simulink model "dsp48_firs_tb"  (Simulink 7.0)
settings: Solver=ode45  StartTime=0.0  StopTime=200  RelTol=1e-3
PreLoadFcn:
  | fir_setup_v1
StartFcn:
  | fir_setup_v1
undefined symbols (not defined in the file): A, B, C, coef, P, PCIN
libraries: xbsIndex_r4 x229, simulink x10, xbsCopyrightNotice_r4 x1, dspsrcs4 x1
(part 2 of 3)

== system dsp48_firs_tb/FIR_T1_foldx4/dsp48_1 ==
  note: Folded FIR Type1 Tap #1
  note: Tap1 - Parallel Type1 FIR filter
      | - DSP48 operation is the  function P=C+ A*B.
      | - Output routed over PCOUT.
      | - All The DSP48 internal pipeline registers are used
      | - The BCIN-BCOUT cascade is not used
      |    since larger delays are requred between stages than 2 delays
      | - The B input is configured to use 1 latency register
  ain : Inport  OutDataType=sfix(16)  OutScaling=2^0
  bin : Inport  Port=2  OutDataType=sfix(16)  OutScaling=2^0
  c : Inport  Port=3  OutDataType=sfix(16)  OutScaling=2^0
  Constant : xbsIndex_r4/Constant  arith_type=DSP48 Instruction  const=1  n_bits=1  bin_pt=0  explicit_period=off  period=1  equ=P=C+(A*B)  opselect=C + A*B  inp2=PCIN>>17  opr=+  inp1=P  carry=CIN  dbl_ovrd=off  block_type=constant
      settings: block_version=VER_STRING_GOES_HERE
  DSP2 : xbsIndex_r4/DSP48  use_b=Direct from B Port  use_op=on  use_creg=on  use_pcin=off  use_pcout=on  use_bcout=off  rst_all=off  en_all=off  pipeline_a=1  pipeline_b=1  pipeline_c=on  pipeline_p=on  pipeline_mult=on  pipeline_opmode=on  pipeline_sub=on  pipeline_carryin=on  pipeline_carryinsel=on  rst_a=off  rst_b=off  rst_c=off  rst_mult=off  rst_p=off  rst_carry_in=off  rst_ctrl=off  en_a=off  en_b=off  en_c=off  en_mult=off  en_p=off  en_carry_in=off  en_ctrl=off  dbl_ovrd=off  use_synth_model=off  xl_useadderonly=off  block_type=dsp48
      settings: xl_use_area=on  xl_area=[0, 0, 0, 0, 0, 0, 0]  block_version=VER_STRING_GOES_HERE
  Terminator1 : Terminator
  pcout : Outport  OutDataType=sfix(16)  OutScaling=2^0
  wires:
  ain/1 -> DSP2/1
  c/1 -> DSP2/3
  bin/1 -> DSP2/2
  DSP2/1 -> Terminator1/1
  DSP2/2 -> pcout/1
  Constant/1 -> DSP2/4

== system dsp48_firs_tb/FIR_T1_foldx4/dsp48_2 ==
  note: Tap2 - Parallel Type1 FIR filter
      | - DSP48 operation is the  function P=PCIN + A*B.
      | - Uses PCIN-PCOUT cascade
      | - All The DSP48 internal pipeline registers are used
      | - The BCIN-BCOUT cascade is not used
      |    since more than 2 delays are requred between stages
      | - The B input is configured to use 1 latency register
  note: Folded FIR Type1 Tap #2:n-1
  ain : Inport  OutDataType=sfix(16)  OutScaling=2^0
  bin : Inport  Port=2  OutDataType=sfix(16)  OutScaling=2^0
  pcin : Inport  Port=3  OutDataType=sfix(16)  OutScaling=2^0
  Constant : xbsIndex_r4/Constant  arith_type=DSP48 Instruction  const=1  n_bits=1  bin_pt=0  explicit_period=off  period=1  equ=P=PCIN+(A*B)  opselect=PCIN + A*B  inp2=PCIN>>17  opr=+  inp1=P  carry=CIN  dbl_ovrd=off  block_type=constant
      settings: block_version=VER_STRING_GOES_HERE
  DSP2 : xbsIndex_r4/DSP48  use_b=Direct from B Port  use_op=on  use_creg=off  use_pcin=on  use_pcout=on  use_bcout=off  rst_all=off  en_all=off  pipeline_a=1  pipeline_b=1  pipeline_c=on  pipeline_p=on  pipeline_mult=on  pipeline_opmode=on  pipeline_sub=on  pipeline_carryin=on  pipeline_carryinsel=on  rst_a=off  rst_b=off  rst_c=off  rst_mult=off  rst_p=off  rst_carry_in=off  rst_ctrl=off  en_a=off  en_b=off  en_c=off  en_mult=off  en_p=off  en_carry_in=off  en_ctrl=off  dbl_ovrd=off  use_synth_model=off  xl_useadderonly=off  block_type=dsp48
      settings: xl_use_area=on  xl_area=[0, 0, 0, 0, 0, 0, 0]  block_version=VER_STRING_GOES_HERE
  Terminator1 : Terminator
  pcout : Outport  OutDataType=sfix(16)  OutScaling=2^0
  wires:
  bin/1 -> DSP2/2
  ain/1 -> DSP2/1
  DSP2/2 -> pcout/1
  DSP2/1 -> Terminator1/1
  pcin/1 -> DSP2/3
  Constant/1 -> DSP2/4

== system dsp48_firs_tb/FIR_T1_foldx4/dsp48_3 ==
  note: Folded FIR Type1 Tap #2:n-1
  note: Tap2 - Parallel Type1 FIR filter
      | - DSP48 operation is the  function P=PCIN + A*B.
      | - Uses PCIN-PCOUT cascade
      | - All The DSP48 internal pipeline registers are used
      | - The BCIN-BCOUT cascade is not used
      |    since more than 2 delays are requred between stages
      | - The B input is configured to use 1 latency register
  ain : Inport  OutDataType=sfix(16)  OutScaling=2^0
  bin : Inport  Port=2  OutDataType=sfix(16)  OutScaling=2^0
  pcin : Inport  Port=3  OutDataType=sfix(16)  OutScaling=2^0
  Constant : xbsIndex_r4/Constant  arith_type=DSP48 Instruction  const=1  n_bits=1  bin_pt=0  explicit_period=off  period=1  equ=P=PCIN+(A*B)  opselect=PCIN + A*B  inp2=PCIN>>17  opr=+  inp1=P  carry=CIN  dbl_ovrd=off  block_type=constant
      settings: block_version=VER_STRING_GOES_HERE
  DSP2 : xbsIndex_r4/DSP48  use_b=Direct from B Port  use_op=on  use_creg=off  use_pcin=on  use_pcout=on  use_bcout=off  rst_all=off  en_all=off  pipeline_a=1  pipeline_b=1  pipeline_c=on  pipeline_p=on  pipeline_mult=on  pipeline_opmode=on  pipeline_sub=on  pipeline_carryin=on  pipeline_carryinsel=on  rst_a=off  rst_b=off  rst_c=off  rst_mult=off  rst_p=off  rst_carry_in=off  rst_ctrl=off  en_a=off  en_b=off  en_c=off  en_mult=off  en_p=off  en_carry_in=off  en_ctrl=off  dbl_ovrd=off  use_synth_model=off  xl_useadderonly=off  block_type=dsp48
      settings: xl_use_area=on  xl_area=[0, 0, 0, 0, 0, 0, 0]  block_version=VER_STRING_GOES_HERE
  Terminator1 : Terminator
  pcout : Outport  OutDataType=sfix(16)  OutScaling=2^0
  wires:
  Constant/1 -> DSP2/4
  pcin/1 -> DSP2/3
  DSP2/1 -> Terminator1/1
  DSP2/2 -> pcout/1
  ain/1 -> DSP2/1
  bin/1 -> DSP2/2

== system dsp48_firs_tb/FIR_T1_foldx4/dsp48_4 ==
  note: Tap2 - Parallel Type1 FIR filter
      | - DSP48 operation is the  function P=PCIN + A*B.
      | - Uses PCIN-PCOUT cascade
      | - All The DSP48 internal pipeline registers are used
      | - The BCIN-BCOUT cascade is not used
      |    since more than 2 delays are requred between stages
      | - The B input is configured to use 1 latency register
  note: Folded FIR Type1 Tap #2:n-1
  ain : Inport  OutDataType=sfix(16)  OutScaling=2^0
  bin : Inport  Port=2  OutDataType=sfix(16)  OutScaling=2^0
  pcin : Inport  Port=3  OutDataType=sfix(16)  OutScaling=2^0
  Constant : xbsIndex_r4/Constant  arith_type=DSP48 Instruction  const=1  n_bits=1  bin_pt=0  explicit_period=off  period=1  equ=P=PCIN+(A*B)  opselect=PCIN + A*B  inp2=PCIN>>17  opr=+  inp1=P  carry=CIN  dbl_ovrd=off  block_type=constant
      settings: block_version=VER_STRING_GOES_HERE
  DSP2 : xbsIndex_r4/DSP48  use_b=Direct from B Port  use_op=on  use_creg=off  use_pcin=on  use_pcout=on  use_bcout=off  rst_all=off  en_all=off  pipeline_a=1  pipeline_b=1  pipeline_c=on  pipeline_p=on  pipeline_mult=on  pipeline_opmode=on  pipeline_sub=on  pipeline_carryin=on  pipeline_carryinsel=on  rst_a=off  rst_b=off  rst_c=off  rst_mult=off  rst_p=off  rst_carry_in=off  rst_ctrl=off  en_a=off  en_b=off  en_c=off  en_mult=off  en_p=off  en_carry_in=off  en_ctrl=off  dbl_ovrd=off  use_synth_model=off  xl_useadderonly=off  block_type=dsp48
      settings: xl_use_area=on  xl_area=[0, 0, 0, 0, 0, 0, 0]  block_version=VER_STRING_GOES_HERE
  Terminator1 : Terminator
  pcout : Outport  OutDataType=sfix(16)  OutScaling=2^0
  wires:
  bin/1 -> DSP2/2
  ain/1 -> DSP2/1
  DSP2/2 -> pcout/1
  DSP2/1 -> Terminator1/1
  pcin/1 -> DSP2/3
  Constant/1 -> DSP2/4

== system dsp48_firs_tb/FIR_T1_foldx4/dsp48_5 ==
  note: Accumulate (ACC)
  note: ACC-  Accumulate Block
      | - DSP48 operation is one of two functions
      |   load:  P= PCIN, .
      |   accumulate: P=P+PCIN
      | - Output routed over P.
      | - All The DSP48 internal pipeline registers are used
      | - DSP48 is used because LUT based adders will not hit speed.
  pcin : Inport  OutDataType=sfix(16)  OutScaling=2^0
  load : Inport  Port=2  OutDataType=sfix(16)  OutScaling=2^0
  Constant : xbsIndex_r4/Constant  arith_type=DSP48 Instruction  const=1  n_bits=1  bin_pt=0  explicit_period=off  period=1  equ=P=PCIN+(P)  opselect=Custom  inp2=PCIN  opr=+  inp1=P  carry=0  dbl_ovrd=off  block_type=constant
      settings: block_version=VER_STRING_GOES_HERE
  Constant1 : xbsIndex_r4/Constant  arith_type=Signed (2's comp)  const=0  n_bits=18  bin_pt=0  explicit_period=on  period=1/4  equ=P=C  opselect=C  inp2=PCIN>>17  opr=+  inp1=P  carry=CIN  dbl_ovrd=off  block_type=constant
      settings: block_version=VER_STRING_GOES_HERE
  Constant2 : xbsIndex_r4/Constant  arith_type=Signed (2's comp)  const=0  n_bits=18  bin_pt=0  explicit_period=on  period=1/4  equ=P=C  opselect=C  inp2=PCIN>>17  opr=+  inp1=P  carry=CIN  dbl_ovrd=off  block_type=constant
      settings: block_version=VER_STRING_GOES_HERE
  Constant3 : xbsIndex_r4/Constant  arith_type=DSP48 Instruction  const=1  n_bits=1  bin_pt=0  explicit_period=off  period=1  equ=P=PCIN  opselect=Custom  inp2=PCIN  opr=+  inp1=0  carry=0  dbl_ovrd=off  block_type=constant
      settings: block_version=VER_STRING_GOES_HERE
  DSP48 : xbsIndex_r4/DSP48  use_b=Direct from B Port  use_op=on  use_creg=off  use_pcin=on  use_pcout=off  use_bcout=off  rst_all=off  en_all=off  pipeline_a=1  pipeline_b=1  pipeline_c=on  pipeline_p=on  pipeline_mult=on  pipeline_opmode=on  pipeline_sub=on  pipeline_carryin=on  pipeline_carryinsel=on  rst_a=off  rst_b=off  rst_c=off  rst_mult=off  rst_p=off  rst_carry_in=off  rst_ctrl=off  en_a=off  en_b=off  en_c=off  en_mult=off  en_p=off  en_carry_in=off  en_ctrl=off  dbl_ovrd=off  use_synth_model=off  xl_useadderonly=off  block_type=dsp48
      settings: xl_use_area=on  xl_area=[0, 0, 0, 0, 0, 0, 0]  block_version=VER_STRING_GOES_HERE
  Mux1 : xbsIndex_r4/Mux  inputs=2  en=off  latency=0  precision=Full  arith_type=Unsigned  n_bits=48  bin_pt=0  quantization=Truncate  overflow=Wrap  dbl_ovrd=off  block_type=mux
      settings: xl_area=[0, 0, 0, 0, 0, 0, 0]  block_version=VER_STRING_GOES_HERE
  out : Outport  OutDataType=sfix(16)  OutScaling=2^0
  wires:
  Constant2/1 -> DSP48/2
  Constant1/1 -> DSP48/1
  DSP48/1 -> out/1
  load/1 -> Mux1/1
  pcin/1 -> DSP48/3
  Mux1/1 -> DSP48/4
  Constant3/1 -> Mux1/3
  Constant/1 -> Mux1/2

== system dsp48_firs_tb/FIR_T1x16/fir_next1 ==
  note: Tap1 - Parallel Type1 FIR filter
      | - DSP48 operation is the  function P=PCIN + A*B.
      | - Output routed over PCOUT.
      | - All The DSP48 internal pipeline registers are used
      | - The BCIN-BCOUT cascade is used
      | - The B input is configured to use 2 latency registers
  note: Parallel FIR Type2 Tap #2:n-1
  ain : Inport  OutDataType=sfix(16)  OutScaling=2^0
  bcin : Inport  Port=2  OutDataType=sfix(16)  OutScaling=2^0
  pcin : Inport  Port=3  OutDataType=sfix(16)  OutScaling=2^0
  Constant : xbsIndex_r4/Constant  arith_type=DSP48 Instruction  const=1  n_bits=1  bin_pt=0  explicit_period=off  period=1  equ=P=PCIN+(A*B)  opselect=PCIN + A*B  inp2=PCIN>>17  opr=+  inp1=P  carry=CIN  dbl_ovrd=off  block_type=constant
      settings: block_version=VER_STRING_GOES_HERE
  DSP48 : xbsIndex_r4/DSP48  use_b=Cascaded from BCIN Port  use_op=on  use_creg=off  use_pcin=on  use_pcout=on  use_bcout=on  rst_all=off  en_all=off  pipeline_a=1  pipeline_b=2  pipeline_c=on  pipeline_p=on  pipeline_mult=on  pipeline_opmode=on  pipeline_sub=on  pipeline_carryin=on  pipeline_carryinsel=on  rst_a=off  rst_b=off  rst_c=off  rst_mult=off  rst_p=off  rst_carry_in=off  rst_ctrl=off  en_a=off  en_b=off  en_c=off  en_mult=off  en_p=off  en_carry_in=off  en_ctrl=off  dbl_ovrd=off  use_synth_model=off  xl_useadderonly=off  block_type=dsp48
      settings: xl_use_area=on  xl_area=[0, 0, 0, 0, 0, 0, 0]  block_version=VER_STRING_GOES_HERE
  Terminator1 : Terminator
  bcout : Outport  OutDataType=sfix(16)  OutScaling=2^0
  pcout : Outport  Port=2  OutDataType=sfix(16)  OutScaling=2^0
  wires:
  bcin/1 -> DSP48/2
  ain/1 -> DSP48/1
  DSP48/3 -> pcout/1
  DSP48/2 -> bcout/1
  DSP48/1 -> Terminator1/1
  pcin/1 -> DSP48/3
  Constant/1 -> DSP48/4

== system dsp48_firs_tb/FIR_T1x16/fir_next10 ==
  note: Parallel FIR Type2 Tap #2:n-1
  note: Tap1 - Parallel Type1 FIR filter
      | - DSP48 operation is the  function P=PCIN + A*B.
      | - Output routed over PCOUT.
      | - All The DSP48 internal pipeline registers are used
      | - The BCIN-BCOUT cascade is used
      | - The B input is configured to use 2 latency registers
  ain : Inport  OutDataType=sfix(16)  OutScaling=2^0
  bcin : Inport  Port=2  OutDataType=sfix(16)  OutScaling=2^0
  pcin : Inport  Port=3  OutDataType=sfix(16)  OutScaling=2^0
  Constant : xbsIndex_r4/Constant  arith_type=DSP48 Instruction  const=1  n_bits=1  bin_pt=0  explicit_period=off  period=1  equ=P=PCIN+(A*B)  opselect=PCIN + A*B  inp2=PCIN>>17  opr=+  inp1=P  carry=CIN  dbl_ovrd=off  block_type=constant
      settings: block_version=VER_STRING_GOES_HERE
  DSP48 : xbsIndex_r4/DSP48  use_b=Cascaded from BCIN Port  use_op=on  use_creg=off  use_pcin=on  use_pcout=on  use_bcout=on  rst_all=off  en_all=off  pipeline_a=1  pipeline_b=2  pipeline_c=on  pipeline_p=on  pipeline_mult=on  pipeline_opmode=on  pipeline_sub=on  pipeline_carryin=on  pipeline_carryinsel=on  rst_a=off  rst_b=off  rst_c=off  rst_mult=off  rst_p=off  rst_carry_in=off  rst_ctrl=off  en_a=off  en_b=off  en_c=off  en_mult=off  en_p=off  en_carry_in=off  en_ctrl=off  dbl_ovrd=off  use_synth_model=off  xl_useadderonly=off  block_type=dsp48
      settings: xl_use_area=on  xl_area=[0, 0, 0, 0, 0, 0, 0]  block_version=VER_STRING_GOES_HERE
  Terminator1 : Terminator
  bcout : Outport  OutDataType=sfix(16)  OutScaling=2^0
  pcout : Outport  Port=2  OutDataType=sfix(16)  OutScaling=2^0
  wires:
  Constant/1 -> DSP48/4
  pcin/1 -> DSP48/3
  DSP48/1 -> Terminator1/1
  DSP48/2 -> bcout/1
  DSP48/3 -> pcout/1
  ain/1 -> DSP48/1
  bcin/1 -> DSP48/2

== system dsp48_firs_tb/FIR_T1x16/fir_next11 ==
  note: Tap1 - Parallel Type1 FIR filter
      | - DSP48 operation is the  function P=PCIN + A*B.
      | - Output routed over PCOUT.
      | - All The DSP48 internal pipeline registers are used
      | - The BCIN-BCOUT cascade is used
      | - The B input is configured to use 2 latency registers
  note: Parallel FIR Type2 Tap #2:n-1
  ain : Inport  OutDataType=sfix(16)  OutScaling=2^0
  bcin : Inport  Port=2  OutDataType=sfix(16)  OutScaling=2^0
  pcin : Inport  Port=3  OutDataType=sfix(16)  OutScaling=2^0
  Constant : xbsIndex_r4/Constant  arith_type=DSP48 Instruction  const=1  n_bits=1  bin_pt=0  explicit_period=off  period=1  equ=P=PCIN+(A*B)  opselect=PCIN + A*B  inp2=PCIN>>17  opr=+  inp1=P  carry=CIN  dbl_ovrd=off  block_type=constant
      settings: block_version=VER_STRING_GOES_HERE
  DSP48 : xbsIndex_r4/DSP48  use_b=Cascaded from BCIN Port  use_op=on  use_creg=off  use_pcin=on  use_pcout=on  use_bcout=on  rst_all=off  en_all=off  pipeline_a=1  pipeline_b=2  pipeline_c=on  pipeline_p=on  pipeline_mult=on  pipeline_opmode=on  pipeline_sub=on  pipeline_carryin=on  pipeline_carryinsel=on  rst_a=off  rst_b=off  rst_c=off  rst_mult=off  rst_p=off  rst_carry_in=off  rst_ctrl=off  en_a=off  en_b=off  en_c=off  en_mult=off  en_p=off  en_carry_in=off  en_ctrl=off  dbl_ovrd=off  use_synth_model=off  xl_useadderonly=off  block_type=dsp48
      settings: xl_use_area=on  xl_area=[0, 0, 0, 0, 0, 0, 0]  block_version=VER_STRING_GOES_HERE
  Terminator1 : Terminator
  bcout : Outport  OutDataType=sfix(16)  OutScaling=2^0
  pcout : Outport  Port=2  OutDataType=sfix(16)  OutScaling=2^0
  wires:
  bcin/1 -> DSP48/2
  ain/1 -> DSP48/1
  DSP48/3 -> pcout/1
  DSP48/2 -> bcout/1
  DSP48/1 -> Terminator1/1
  pcin/1 -> DSP48/3
  Constant/1 -> DSP48/4

== system dsp48_firs_tb/FIR_T1x16/fir_next12 ==
  note: Parallel FIR Type2 Tap #2:n-1
  note: Tap1 - Parallel Type1 FIR filter
      | - DSP48 operation is the  function P=PCIN + A*B.
      | - Output routed over PCOUT.
      | - All The DSP48 internal pipeline registers are used
      | - The BCIN-BCOUT cascade is used
      | - The B input is configured to use 2 latency registers
  ain : Inport  OutDataType=sfix(16)  OutScaling=2^0
  bcin : Inport  Port=2  OutDataType=sfix(16)  OutScaling=2^0
  pcin : Inport  Port=3  OutDataType=sfix(16)  OutScaling=2^0
  Constant : xbsIndex_r4/Constant  arith_type=DSP48 Instruction  const=1  n_bits=1  bin_pt=0  explicit_period=off  period=1  equ=P=PCIN+(A*B)  opselect=PCIN + A*B  inp2=PCIN>>17  opr=+  inp1=P  carry=CIN  dbl_ovrd=off  block_type=constant
      settings: block_version=VER_STRING_GOES_HERE
  DSP48 : xbsIndex_r4/DSP48  use_b=Cascaded from BCIN Port  use_op=on  use_creg=off  use_pcin=on  use_pcout=on  use_bcout=on  rst_all=off  en_all=off  pipeline_a=1  pipeline_b=2  pipeline_c=on  pipeline_p=on  pipeline_mult=on  pipeline_opmode=on  pipeline_sub=on  pipeline_carryin=on  pipeline_carryinsel=on  rst_a=off  rst_b=off  rst_c=off  rst_mult=off  rst_p=off  rst_carry_in=off  rst_ctrl=off  en_a=off  en_b=off  en_c=off  en_mult=off  en_p=off  en_carry_in=off  en_ctrl=off  dbl_ovrd=off  use_synth_model=off  xl_useadderonly=off  block_type=dsp48
      settings: xl_use_area=on  xl_area=[0, 0, 0, 0, 0, 0, 0]  block_version=VER_STRING_GOES_HERE
  Terminator1 : Terminator
  bcout : Outport  OutDataType=sfix(16)  OutScaling=2^0
  pcout : Outport  Port=2  OutDataType=sfix(16)  OutScaling=2^0
  wires:
  Constant/1 -> DSP48/4
  pcin/1 -> DSP48/3
  DSP48/1 -> Terminator1/1
  DSP48/2 -> bcout/1
  DSP48/3 -> pcout/1
  ain/1 -> DSP48/1
  bcin/1 -> DSP48/2

== system dsp48_firs_tb/FIR_T1x16/fir_next13 ==
  note: Tap1 - Parallel Type1 FIR filter
      | - DSP48 operation is the  function P=PCIN + A*B.
      | - Output routed over PCOUT.
      | - All The DSP48 internal pipeline registers are used
      | - The BCIN-BCOUT cascade is used
      | - The B input is configured to use 2 latency registers
  note: Parallel FIR Type2 Tap #2:n-1
  ain : Inport  OutDataType=sfix(16)  OutScaling=2^0
  bcin : Inport  Port=2  OutDataType=sfix(16)  OutScaling=2^0
  pcin : Inport  Port=3  OutDataType=sfix(16)  OutScaling=2^0
  Constant : xbsIndex_r4/Constant  arith_type=DSP48 Instruction  const=1  n_bits=1  bin_pt=0  explicit_period=off  period=1  equ=P=PCIN+(A*B)  opselect=PCIN + A*B  inp2=PCIN>>17  opr=+  inp1=P  carry=CIN  dbl_ovrd=off  block_type=constant
      settings: block_version=VER_STRING_GOES_HERE
  DSP48 : xbsIndex_r4/DSP48  use_b=Cascaded from BCIN Port  use_op=on  use_creg=off  use_pcin=on  use_pcout=on  use_bcout=on  rst_all=off  en_all=off  pipeline_a=1  pipeline_b=2  pipeline_c=on  pipeline_p=on  pipeline_mult=on  pipeline_opmode=on  pipeline_sub=on  pipeline_carryin=on  pipeline_carryinsel=on  rst_a=off  rst_b=off  rst_c=off  rst_mult=off  rst_p=off  rst_carry_in=off  rst_ctrl=off  en_a=off  en_b=off  en_c=off  en_mult=off  en_p=off  en_carry_in=off  en_ctrl=off  dbl_ovrd=off  use_synth_model=off  xl_useadderonly=off  block_type=dsp48
      settings: xl_use_area=on  xl_area=[0, 0, 0, 0, 0, 0, 0]  block_version=VER_STRING_GOES_HERE
  Terminator1 : Terminator
  bcout : Outport  OutDataType=sfix(16)  OutScaling=2^0
  pcout : Outport  Port=2  OutDataType=sfix(16)  OutScaling=2^0
  wires:
  bcin/1 -> DSP48/2
  ain/1 -> DSP48/1
  DSP48/3 -> pcout/1
  DSP48/2 -> bcout/1
  DSP48/1 -> Terminator1/1
  pcin/1 -> DSP48/3
  Constant/1 -> DSP48/4

== system dsp48_firs_tb/FIR_T1x16/fir_next14 ==
  note: Parallel FIR Type2 Tap #2:n-1
  note: Tap1 - Parallel Type1 FIR filter
      | - DSP48 operation is the  function P=PCIN + A*B.
      | - Output routed over PCOUT.
      | - All The DSP48 internal pipeline registers are used
      | - The BCIN-BCOUT cascade is used
      | - The B input is configured to use 2 latency registers
  ain : Inport  OutDataType=sfix(16)  OutScaling=2^0
  bcin : Inport  Port=2  OutDataType=sfix(16)  OutScaling=2^0
  pcin : Inport  Port=3  OutDataType=sfix(16)  OutScaling=2^0
  Constant : xbsIndex_r4/Constant  arith_type=DSP48 Instruction  const=1  n_bits=1  bin_pt=0  explicit_period=off  period=1  equ=P=PCIN+(A*B)  opselect=PCIN + A*B  inp2=PCIN>>17  opr=+  inp1=P  carry=CIN  dbl_ovrd=off  block_type=constant
      settings: block_version=VER_STRING_GOES_HERE
  DSP48 : xbsIndex_r4/DSP48  use_b=Cascaded from BCIN Port  use_op=on  use_creg=off  use_pcin=on  use_pcout=on  use_bcout=on  rst_all=off  en_all=off  pipeline_a=1  pipeline_b=2  pipeline_c=on  pipeline_p=on  pipeline_mult=on  pipeline_opmode=on  pipeline_sub=on  pipeline_carryin=on  pipeline_carryinsel=on  rst_a=off  rst_b=off  rst_c=off  rst_mult=off  rst_p=off  rst_carry_in=off  rst_ctrl=off  en_a=off  en_b=off  en_c=off  en_mult=off  en_p=off  en_carry_in=off  en_ctrl=off  dbl_ovrd=off  use_synth_model=off  xl_useadderonly=off  block_type=dsp48
      settings: xl_use_area=on  xl_area=[0, 0, 0, 0, 0, 0, 0]  block_version=VER_STRING_GOES_HERE
  Terminator1 : Terminator
  bcout : Outport  OutDataType=sfix(16)  OutScaling=2^0
  pcout : Outport  Port=2  OutDataType=sfix(16)  OutScaling=2^0
  wires:
  Constant/1 -> DSP48/4
  pcin/1 -> DSP48/3
  DSP48/1 -> Terminator1/1
  DSP48/2 -> bcout/1
  DSP48/3 -> pcout/1
  ain/1 -> DSP48/1
  bcin/1 -> DSP48/2

== system dsp48_firs_tb/FIR_T1x16/fir_next15 ==
  note: Tap1 - Parallel Type1 FIR filter
      | - DSP48 operation is the  function P=PCIN + A*B.
      | - Output from C
      | - All The DSP48 internal pipeline registers are used
      | - The BCIN-BCOUT cascade is used
      | - The B input is configured to use 2 latency registers
  note: Parallel FIR Type2 Tap #n
  ain : Inport  OutDataType=sfix(16)  OutScaling=2^0
  bcin : Inport  Port=2  OutDataType=sfix(16)  OutScaling=2^0
  pcin : Inport  Port=3  OutDataType=sfix(16)  OutScaling=2^0
  Constant : xbsIndex_r4/Constant  arith_type=DSP48 Instruction  const=1  n_bits=1  bin_pt=0  explicit_period=off  period=1  equ=P=PCIN+(A*B)  opselect=PCIN + A*B  inp2=PCIN>>17  opr=+  inp1=P  carry=CIN  dbl_ovrd=off  block_type=constant
      settings: block_version=VER_STRING_GOES_HERE
  DSP48 : xbsIndex_r4/DSP48  use_b=Cascaded from BCIN Port  use_op=on  use_creg=off  use_pcin=on  use_pcout=off  use_bcout=off  rst_all=off  en_all=off  pipeline_a=1  pipeline_b=2  pipeline_c=on  pipeline_p=on  pipeline_mult=on  pipeline_opmode=on  pipeline_sub=on  pipeline_carryin=on  pipeline_carryinsel=on  rst_a=off  rst_b=off  rst_c=off  rst_mult=off  rst_p=off  rst_carry_in=off  rst_ctrl=off  en_a=off  en_b=off  en_c=off  en_mult=off  en_p=off  en_carry_in=off  en_ctrl=off  dbl_ovrd=off  use_synth_model=off  xl_useadderonly=off  block_type=dsp48
      settings: xl_use_area=on  xl_area=[0, 0, 0, 0, 0, 0, 0]  block_version=VER_STRING_GOES_HERE
  p : Outport  OutDataType=sfix(16)  OutScaling=2^0
  wires:
  bcin/1 -> DSP48/2
  ain/1 -> DSP48/1
  DSP48/1 -> p/1
  pcin/1 -> DSP48/3
  Constant/1 -> DSP48/4

== system dsp48_firs_tb/FIR_T1x16/fir_next2 ==
  note: Parallel FIR Type2 Tap #2:n-1
  note: Tap1 - Parallel Type1 FIR filter
      | - DSP48 operation is the  function P=PCIN + A*B.
      | - Output routed over PCOUT.
      | - All The DSP48 internal pipeline registers are used
      | - The BCIN-BCOUT cascade is used
      | - The B input is configured to use 2 latency registers
  ain : Inport  OutDataType=sfix(16)  OutScaling=2^0
  bcin : Inport  Port=2  OutDataType=sfix(16)  OutScaling=2^0
  pcin : Inport  Port=3  OutDataType=sfix(16)  OutScaling=2^0
  Constant : xbsIndex_r4/Constant  arith_type=DSP48 Instruction  const=1  n_bits=1  bin_pt=0  explicit_period=off  period=1  equ=P=PCIN+(A*B)  opselect=PCIN + A*B  inp2=PCIN>>17  opr=+  inp1=P  carry=CIN  dbl_ovrd=off  block_type=constant
      settings: block_version=VER_STRING_GOES_HERE
  DSP48 : xbsIndex_r4/DSP48  use_b=Cascaded from BCIN Port  use_op=on  use_creg=off  use_pcin=on  use_pcout=on  use_bcout=on  rst_all=off  en_all=off  pipeline_a=1  pipeline_b=2  pipeline_c=on  pipeline_p=on  pipeline_mult=on  pipeline_opmode=on  pipeline_sub=on  pipeline_carryin=on  pipeline_carryinsel=on  rst_a=off  rst_b=off  rst_c=off  rst_mult=off  rst_p=off  rst_carry_in=off  rst_ctrl=off  en_a=off  en_b=off  en_c=off  en_mult=off  en_p=off  en_carry_in=off  en_ctrl=off  dbl_ovrd=off  use_synth_model=off  xl_useadderonly=off  block_type=dsp48
      settings: xl_use_area=on  xl_area=[0, 0, 0, 0, 0, 0, 0]  block_version=VER_STRING_GOES_HERE
  Terminator1 : Terminator
  bcout : Outport  OutDataType=sfix(16)  OutScaling=2^0
  pcout : Outport  Port=2  OutDataType=sfix(16)  OutScaling=2^0
  wires:
  Constant/1 -> DSP48/4
  pcin/1 -> DSP48/3
  DSP48/1 -> Terminator1/1
  DSP48/2 -> bcout/1
  DSP48/3 -> pcout/1
  ain/1 -> DSP48/1
  bcin/1 -> DSP48/2

== system dsp48_firs_tb/FIR_T1x16/fir_next3 ==
  note: Tap1 - Parallel Type1 FIR filter
      | - DSP48 operation is the  function P=PCIN + A*B.
      | - Output routed over PCOUT.
      | - All The DSP48 internal pipeline registers are used
      | - The BCIN-BCOUT cascade is used
      | - The B input is configured to use 2 latency registers
  note: Parallel FIR Type2 Tap #2:n-1
  ain : Inport  OutDataType=sfix(16)  OutScaling=2^0
  bcin : Inport  Port=2  OutDataType=sfix(16)  OutScaling=2^0
  pcin : Inport  Port=3  OutDataType=sfix(16)  OutScaling=2^0
  Constant : xbsIndex_r4/Constant  arith_type=DSP48 Instruction  const=1  n_bits=1  bin_pt=0  explicit_period=off  period=1  equ=P=PCIN+(A*B)  opselect=PCIN + A*B  inp2=PCIN>>17  opr=+  inp1=P  carry=CIN  dbl_ovrd=off  block_type=constant
      settings: block_version=VER_STRING_GOES_HERE
  DSP48 : xbsIndex_r4/DSP48  use_b=Cascaded from BCIN Port  use_op=on  use_creg=off  use_pcin=on  use_pcout=on  use_bcout=on  rst_all=off  en_all=off  pipeline_a=1  pipeline_b=2  pipeline_c=on  pipeline_p=on  pipeline_mult=on  pipeline_opmode=on  pipeline_sub=on  pipeline_carryin=on  pipeline_carryinsel=on  rst_a=off  rst_b=off  rst_c=off  rst_mult=off  rst_p=off  rst_carry_in=off  rst_ctrl=off  en_a=off  en_b=off  en_c=off  en_mult=off  en_p=off  en_carry_in=off  en_ctrl=off  dbl_ovrd=off  use_synth_model=off  xl_useadderonly=off  block_type=dsp48
      settings: xl_use_area=on  xl_area=[0, 0, 0, 0, 0, 0, 0]  block_version=VER_STRING_GOES_HERE
  Terminator1 : Terminator
  bcout : Outport  OutDataType=sfix(16)  OutScaling=2^0
  pcout : Outport  Port=2  OutDataType=sfix(16)  OutScaling=2^0
  wires:
  bcin/1 -> DSP48/2
  ain/1 -> DSP48/1
  DSP48/3 -> pcout/1
  DSP48/2 -> bcout/1
  DSP48/1 -> Terminator1/1
  pcin/1 -> DSP48/3
  Constant/1 -> DSP48/4

== system dsp48_firs_tb/FIR_T1x16/fir_next4 ==
  note: Parallel FIR Type2 Tap #2:n-1
  note: Tap1 - Parallel Type1 FIR filter
      | - DSP48 operation is the  function P=PCIN + A*B.
      | - Output routed over PCOUT.
      | - All The DSP48 internal pipeline registers are used
      | - The BCIN-BCOUT cascade is used
      | - The B input is configured to use 2 latency registers
  ain : Inport  OutDataType=sfix(16)  OutScaling=2^0
  bcin : Inport  Port=2  OutDataType=sfix(16)  OutScaling=2^0
  pcin : Inport  Port=3  OutDataType=sfix(16)  OutScaling=2^0
  Constant : xbsIndex_r4/Constant  arith_type=DSP48 Instruction  const=1  n_bits=1  bin_pt=0  explicit_period=off  period=1  equ=P=PCIN+(A*B)  opselect=PCIN + A*B  inp2=PCIN>>17  opr=+  inp1=P  carry=CIN  dbl_ovrd=off  block_type=constant
      settings: block_version=VER_STRING_GOES_HERE
  DSP48 : xbsIndex_r4/DSP48  use_b=Cascaded from BCIN Port  use_op=on  use_creg=off  use_pcin=on  use_pcout=on  use_bcout=on  rst_all=off  en_all=off  pipeline_a=1  pipeline_b=2  pipeline_c=on  pipeline_p=on  pipeline_mult=on  pipeline_opmode=on  pipeline_sub=on  pipeline_carryin=on  pipeline_carryinsel=on  rst_a=off  rst_b=off  rst_c=off  rst_mult=off  rst_p=off  rst_carry_in=off  rst_ctrl=off  en_a=off  en_b=off  en_c=off  en_mult=off  en_p=off  en_carry_in=off  en_ctrl=off  dbl_ovrd=off  use_synth_model=off  xl_useadderonly=off  block_type=dsp48
      settings: xl_use_area=on  xl_area=[0, 0, 0, 0, 0, 0, 0]  block_version=VER_STRING_GOES_HERE
  Terminator1 : Terminator
  bcout : Outport  OutDataType=sfix(16)  OutScaling=2^0
  pcout : Outport  Port=2  OutDataType=sfix(16)  OutScaling=2^0
  wires:
  Constant/1 -> DSP48/4
  pcin/1 -> DSP48/3
  DSP48/1 -> Terminator1/1
  DSP48/2 -> bcout/1
  DSP48/3 -> pcout/1
  ain/1 -> DSP48/1
  bcin/1 -> DSP48/2

== system dsp48_firs_tb/FIR_T1x16/fir_next5 ==
  note: Tap1 - Parallel Type1 FIR filter
      | - DSP48 operation is the  function P=PCIN + A*B.
      | - Output routed over PCOUT.
      | - All The DSP48 internal pipeline registers are used
      | - The BCIN-BCOUT cascade is used
      | - The B input is configured to use 2 latency registers
  note: Parallel FIR Type2 Tap #2:n-1
  ain : Inport  OutDataType=sfix(16)  OutScaling=2^0
  bcin : Inport  Port=2  OutDataType=sfix(16)  OutScaling=2^0
  pcin : Inport  Port=3  OutDataType=sfix(16)  OutScaling=2^0
  Constant : xbsIndex_r4/Constant  arith_type=DSP48 Instruction  const=1  n_bits=1  bin_pt=0  explicit_period=off  period=1  equ=P=PCIN+(A*B)  opselect=PCIN + A*B  inp2=PCIN>>17  opr=+  inp1=P  carry=CIN  dbl_ovrd=off  block_type=constant
      settings: block_version=VER_STRING_GOES_HERE
  DSP48 : xbsIndex_r4/DSP48  use_b=Cascaded from BCIN Port  use_op=on  use_creg=off  use_pcin=on  use_pcout=on  use_bcout=on  rst_all=off  en_all=off  pipeline_a=1  pipeline_b=2  pipeline_c=on  pipeline_p=on  pipeline_mult=on  pipeline_opmode=on  pipeline_sub=on  pipeline_carryin=on  pipeline_carryinsel=on  rst_a=off  rst_b=off  rst_c=off  rst_mult=off  rst_p=off  rst_carry_in=off  rst_ctrl=off  en_a=off  en_b=off  en_c=off  en_mult=off  en_p=off  en_carry_in=off  en_ctrl=off  dbl_ovrd=off  use_synth_model=off  xl_useadderonly=off  block_type=dsp48
      settings: xl_use_area=on  xl_area=[0, 0, 0, 0, 0, 0, 0]  block_version=VER_STRING_GOES_HERE
  Terminator1 : Terminator
  bcout : Outport  OutDataType=sfix(16)  OutScaling=2^0
  pcout : Outport  Port=2  OutDataType=sfix(16)  OutScaling=2^0
  wires:
  bcin/1 -> DSP48/2
  ain/1 -> DSP48/1
  DSP48/3 -> pcout/1
  DSP48/2 -> bcout/1
  DSP48/1 -> Terminator1/1
  pcin/1 -> DSP48/3
  Constant/1 -> DSP48/4

== system dsp48_firs_tb/FIR_T1x16/fir_next6 ==
  note: Parallel FIR Type2 Tap #2:n-1
  note: Tap1 - Parallel Type1 FIR filter
      | - DSP48 operation is the  function P=PCIN + A*B.
      | - Output routed over PCOUT.
      | - All The DSP48 internal pipeline registers are used
      | - The BCIN-BCOUT cascade is used
      | - The B input is configured to use 2 latency registers
  ain : Inport  OutDataType=sfix(16)  OutScaling=2^0
  bcin : Inport  Port=2  OutDataType=sfix(16)  OutScaling=2^0
  pcin : Inport  Port=3  OutDataType=sfix(16)  OutScaling=2^0
  Constant : xbsIndex_r4/Constant  arith_type=DSP48 Instruction  const=1  n_bits=1  bin_pt=0  explicit_period=off  period=1  equ=P=PCIN+(A*B)  opselect=PCIN + A*B  inp2=PCIN>>17  opr=+  inp1=P  carry=CIN  dbl_ovrd=off  block_type=constant
      settings: block_version=VER_STRING_GOES_HERE
  DSP48 : xbsIndex_r4/DSP48  use_b=Cascaded from BCIN Port  use_op=on  use_creg=off  use_pcin=on  use_pcout=on  use_bcout=on  rst_all=off  en_all=off  pipeline_a=1  pipeline_b=2  pipeline_c=on  pipeline_p=on  pipeline_mult=on  pipeline_opmode=on  pipeline_sub=on  pipeline_carryin=on  pipeline_carryinsel=on  rst_a=off  rst_b=off  rst_c=off  rst_mult=off  rst_p=off  rst_carry_in=off  rst_ctrl=off  en_a=off  en_b=off  en_c=off  en_mult=off  en_p=off  en_carry_in=off  en_ctrl=off  dbl_ovrd=off  use_synth_model=off  xl_useadderonly=off  block_type=dsp48
      settings: xl_use_area=on  xl_area=[0, 0, 0, 0, 0, 0, 0]  block_version=VER_STRING_GOES_HERE
  Terminator1 : Terminator
  bcout : Outport  OutDataType=sfix(16)  OutScaling=2^0
  pcout : Outport  Port=2  OutDataType=sfix(16)  OutScaling=2^0
  wires:
  Constant/1 -> DSP48/4
  pcin/1 -> DSP48/3
  DSP48/1 -> Terminator1/1
  DSP48/2 -> bcout/1
  DSP48/3 -> pcout/1
  ain/1 -> DSP48/1
  bcin/1 -> DSP48/2

== system dsp48_firs_tb/FIR_T1x16/fir_next7 ==
  note: Tap1 - Parallel Type1 FIR filter
      | - DSP48 operation is the  function P=PCIN + A*B.
      | - Output routed over PCOUT.
      | - All The DSP48 internal pipeline registers are used
      | - The BCIN-BCOUT cascade is used
      | - The B input is configured to use 2 latency registers
  note: Parallel FIR Type2 Tap #2:n-1
  ain : Inport  OutDataType=sfix(16)  OutScaling=2^0
  bcin : Inport  Port=2  OutDataType=sfix(16)  OutScaling=2^0
  pcin : Inport  Port=3  OutDataType=sfix(16)  OutScaling=2^0
  Constant : xbsIndex_r4/Constant  arith_type=DSP48 Instruction  const=1  n_bits=1  bin_pt=0  explicit_period=off  period=1  equ=P=PCIN+(A*B)  opselect=PCIN + A*B  inp2=PCIN>>17  opr=+  inp1=P  carry=CIN  dbl_ovrd=off  block_type=constant
      settings: block_version=VER_STRING_GOES_HERE
  DSP48 : xbsIndex_r4/DSP48  use_b=Cascaded from BCIN Port  use_op=on  use_creg=off  use_pcin=on  use_pcout=on  use_bcout=on  rst_all=off  en_all=off  pipeline_a=1  pipeline_b=2  pipeline_c=on  pipeline_p=on  pipeline_mult=on  pipeline_opmode=on  pipeline_sub=on  pipeline_carryin=on  pipeline_carryinsel=on  rst_a=off  rst_b=off  rst_c=off  rst_mult=off  rst_p=off  rst_carry_in=off  rst_ctrl=off  en_a=off  en_b=off  en_c=off  en_mult=off  en_p=off  en_carry_in=off  en_ctrl=off  dbl_ovrd=off  use_synth_model=off  xl_useadderonly=off  block_type=dsp48
      settings: xl_use_area=on  xl_area=[0, 0, 0, 0, 0, 0, 0]  block_version=VER_STRING_GOES_HERE
  Terminator1 : Terminator
  bcout : Outport  OutDataType=sfix(16)  OutScaling=2^0
  pcout : Outport  Port=2  OutDataType=sfix(16)  OutScaling=2^0
  wires:
  bcin/1 -> DSP48/2
  ain/1 -> DSP48/1
  DSP48/3 -> pcout/1
  DSP48/2 -> bcout/1
  DSP48/1 -> Terminator1/1
  pcin/1 -> DSP48/3
  Constant/1 -> DSP48/4

== system dsp48_firs_tb/FIR_T1x16/fir_next8 ==
  note: Parallel FIR Type2 Tap #2:n-1
  note: Tap1 - Parallel Type1 FIR filter
      | - DSP48 operation is the  function P=PCIN + A*B.
      | - Output routed over PCOUT.
      | - All The DSP48 internal pipeline registers are used
      | - The BCIN-BCOUT cascade is used
      | - The B input is configured to use 2 latency registers
  ain : Inport  OutDataType=sfix(16)  OutScaling=2^0
  bcin : Inport  Port=2  OutDataType=sfix(16)  OutScaling=2^0
  pcin : Inport  Port=3  OutDataType=sfix(16)  OutScaling=2^0
  Constant : xbsIndex_r4/Constant  arith_type=DSP48 Instruction  const=1  n_bits=1  bin_pt=0  explicit_period=off  period=1  equ=P=PCIN+(A*B)  opselect=PCIN + A*B  inp2=PCIN>>17  opr=+  inp1=P  carry=CIN  dbl_ovrd=off  block_type=constant
      settings: block_version=VER_STRING_GOES_HERE
  DSP48 : xbsIndex_r4/DSP48  use_b=Cascaded from BCIN Port  use_op=on  use_creg=off  use_pcin=on  use_pcout=on  use_bcout=on  rst_all=off  en_all=off  pipeline_a=1  pipeline_b=2  pipeline_c=on  pipeline_p=on  pipeline_mult=on  pipeline_opmode=on  pipeline_sub=on  pipeline_carryin=on  pipeline_carryinsel=on  rst_a=off  rst_b=off  rst_c=off  rst_mult=off  rst_p=off  rst_carry_in=off  rst_ctrl=off  en_a=off  en_b=off  en_c=off  en_mult=off  en_p=off  en_carry_in=off  en_ctrl=off  dbl_ovrd=off  use_synth_model=off  xl_useadderonly=off  block_type=dsp48
      settings: xl_use_area=on  xl_area=[0, 0, 0, 0, 0, 0, 0]  block_version=VER_STRING_GOES_HERE
  Terminator1 : Terminator
  bcout : Outport  OutDataType=sfix(16)  OutScaling=2^0
  pcout : Outport  Port=2  OutDataType=sfix(16)  OutScaling=2^0
  wires:
  Constant/1 -> DSP48/4
  pcin/1 -> DSP48/3
  DSP48/1 -> Terminator1/1
  DSP48/2 -> bcout/1
  DSP48/3 -> pcout/1
  ain/1 -> DSP48/1
  bcin/1 -> DSP48/2

== system dsp48_firs_tb/FIR_T1x16/fir_next9 ==
  note: Tap1 - Parallel Type1 FIR filter
      | - DSP48 operation is the  function P=PCIN + A*B.
      | - Output routed over PCOUT.
      | - All The DSP48 internal pipeline registers are used
      | - The BCIN-BCOUT cascade is used
      | - The B input is configured to use 2 latency registers
  note: Parallel FIR Type2 Tap #2:n-1
  ain : Inport  OutDataType=sfix(16)  OutScaling=2^0
  bcin : Inport  Port=2  OutDataType=sfix(16)  OutScaling=2^0
  pcin : Inport  Port=3  OutDataType=sfix(16)  OutScaling=2^0
  Constant : xbsIndex_r4/Constant  arith_type=DSP48 Instruction  const=1  n_bits=1  bin_pt=0  explicit_period=off  period=1  equ=P=PCIN+(A*B)  opselect=PCIN + A*B  inp2=PCIN>>17  opr=+  inp1=P  carry=CIN  dbl_ovrd=off  block_type=constant
      settings: block_version=VER_STRING_GOES_HERE
  DSP48 : xbsIndex_r4/DSP48  use_b=Cascaded from BCIN Port  use_op=on  use_creg=off  use_pcin=on  use_pcout=on  use_bcout=on  rst_all=off  en_all=off  pipeline_a=1  pipeline_b=2  pipeline_c=on  pipeline_p=on  pipeline_mult=on  pipeline_opmode=on  pipeline_sub=on  pipeline_carryin=on  pipeline_carryinsel=on  rst_a=off  rst_b=off  rst_c=off  rst_mult=off  rst_p=off  rst_carry_in=off  rst_ctrl=off  en_a=off  en_b=off  en_c=off  en_mult=off  en_p=off  en_carry_in=off  en_ctrl=off  dbl_ovrd=off  use_synth_model=off  xl_useadderonly=off  block_type=dsp48
      settings: xl_use_area=on  xl_area=[0, 0, 0, 0, 0, 0, 0]  block_version=VER_STRING_GOES_HERE
  Terminator1 : Terminator
  bcout : Outport  OutDataType=sfix(16)  OutScaling=2^0
  pcout : Outport  Port=2  OutDataType=sfix(16)  OutScaling=2^0
  wires:
  bcin/1 -> DSP48/2
  ain/1 -> DSP48/1
  DSP48/3 -> pcout/1
  DSP48/2 -> bcout/1
  DSP48/1 -> Terminator1/1
  pcin/1 -> DSP48/3
  Constant/1 -> DSP48/4

== system dsp48_firs_tb/FIR_T1x16/fir_start ==
  note: Parallel FIR Type1 Tap #1
  note: Tap1 - Parallel Type1 FIR filter
      | - DSP48 operation is the  function P=C+ A*B.
      | - Output routed over PCOUT.
      | - All The DSP48 internal pipeline registers are used
      | - The BCIN-BCOUT cascade is used
      | - The B input is configured to use 2 latency registers
  ain : Inport  OutDataType=sfix(16)  OutScaling=2^0
  bin : Inport  Port=2  OutDataType=sfix(16)  OutScaling=2^0
  c : Inport  Port=3  OutDataType=sfix(16)  OutScaling=2^0
  Constant1 : xbsIndex_r4/Constant  arith_type=DSP48 Instruction  const=1  n_bits=1  bin_pt=0  explicit_period=off  period=1  equ=P=C+(A*B)  opselect=C + A*B  inp2=PCIN>>17  opr=+  inp1=P  carry=CIN  dbl_ovrd=off  block_type=constant
      settings: block_version=VER_STRING_GOES_HERE
  DSP48 : xbsIndex_r4/DSP48  use_b=Direct from B Port  use_op=on  use_creg=on  use_pcin=off  use_pcout=on  use_bcout=on  rst_all=off  en_all=off  pipeline_a=1  pipeline_b=2  pipeline_c=on  pipeline_p=on  pipeline_mult=on  pipeline_opmode=on  pipeline_sub=on  pipeline_carryin=on  pipeline_carryinsel=on  rst_a=off  rst_b=off  rst_c=off  rst_mult=off  rst_p=off  rst_carry_in=off  rst_ctrl=off  en_a=off  en_b=off  en_c=off  en_mult=off  en_p=off  en_carry_in=off  en_ctrl=off  dbl_ovrd=off  use_synth_model=off  xl_useadderonly=off  block_type=dsp48
      settings: xl_use_area=on  xl_area=[0, 0, 0, 0, 0, 0, 0]  block_version=VER_STRING_GOES_HERE
  Terminator1 : Terminator
  bcout : Outport  OutDataType=sfix(16)  OutScaling=2^0
  pcout : Outport  Port=2  OutDataType=sfix(16)  OutScaling=2^0
  wires:
  Constant1/1 -> DSP48/4
  ain/1 -> DSP48/1
  c/1 -> DSP48/3
  bin/1 -> DSP48/2
  DSP48/1 -> Terminator1/1
  DSP48/2 -> bcout/1
  DSP48/3 -> pcout/1

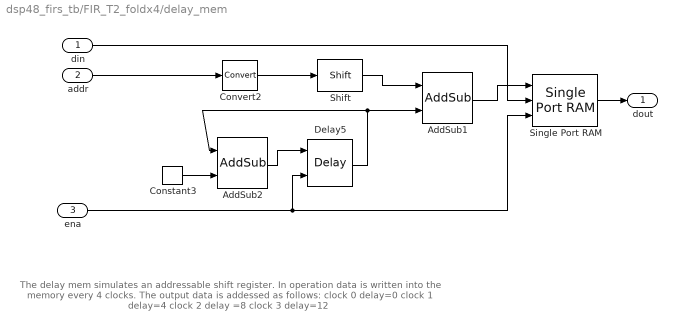
== system dsp48_firs_tb/FIR_T2_foldx4/delay_mem ==
  note: The delay mem simulates an addressable shift register.
      |  In operation data is written into the memory every 4 clocks.
      | The output data is addessed as follows:
      | clock 0   delay=0
      | clock 1   delay=4
      | clock 2  delay =8
      | clock 3  delay=12
  din : Inport  OutDataType=sfix(16)  OutScaling=2^0
  addr : Inport  Port=2  OutDataType=sfix(16)  OutScaling=2^0
  ena : Inport  Port=3  OutDataType=sfix(16)  OutScaling=2^0
  AddSub1 : xbsIndex_r4/AddSub  mode=Subtraction  use_carryin=off  use_carryout=off  en=off  latency=0  precision=User Defined  arith_type=Unsigned  n_bits=4  bin_pt=0  quantization=Truncate  overflow=Wrap  dbl_ovrd=off  use_behavioral_HDL=off  pipelined=off  use_rpm=off  block_type=addsub
      settings: xl_area=[0, 0, 0, 0, 0, 0, 0]  block_version=VER_STRING_GOES_HERE
  AddSub2 : xbsIndex_r4/AddSub  mode=Addition  use_carryin=off  use_carryout=off  en=off  latency=0  precision=User Defined  arith_type=Unsigned  n_bits=4  bin_pt=0  quantization=Truncate  overflow=Wrap  dbl_ovrd=off  use_behavioral_HDL=off  pipelined=off  use_rpm=off  block_type=addsub
      settings: xl_area=[0, 0, 0, 0, 0, 0, 0]  block_version=VER_STRING_GOES_HERE
  Constant3 : xbsIndex_r4/Constant  arith_type=Unsigned  const=1  n_bits=4  bin_pt=0  explicit_period=off  period=1  equ=P=C  opselect=C  inp2=PCIN>>17  opr=+  inp1=P  carry=CIN  dbl_ovrd=off  block_type=constant
      settings: block_version=VER_STRING_GOES_HERE
  Convert2 : xbsIndex_r4/Convert  arith_type=Unsigned  n_bits=4  bin_pt=0  quantization=Truncate  overflow=Wrap  latency=0  dbl_ovrd=off  pipeline=off  block_type=convert
      settings: infoedit=The input is presented at the output after quantization and overflow effects.<P><P>Hardware notes: Additional hardware is used when rounding or saturation is selected and output width is less than the input width.  xl_area=[0, 0, 0, 0, 0, 0, 0]  block_version=VER_STRING_GOES_HERE
  Delay5 : xbsIndex_r4/Delay  en=on  latency=1  dbl_ovrd=off  reg_retiming=off  block_type=delay
      settings: infoedit="Delay line having  configurable length.<P><P>Hardware notes: A delay line is a chain, each link of which is an SRL16 followed by a flip-flop. If register retiming is enabled, the delay line is a chain of flip-flops."  xl_area=[0, 0, 0, 0, 0, 0, 0]  block_version=VER_STRING_GOES_HERE
  Shift : xbsIndex_r4/Shift  shift_dir=Left  shift_bits=2  en=off  latency=0  precision=Full  arith_type="Signed  (2's comp)"  n_bits=8  bin_pt=2  quantization=Truncate  overflow=Wrap  dbl_ovrd=off  block_type=shift
      settings: xl_area=[0, 0, 0, 0, 0, 0, 0]  block_version=VER_STRING_GOES_HERE
  Single Port RAM : xbsIndex_r4/Single Port RAM  depth=16  initVector=0  distributed_mem=Block RAM  write_mode=Read Before Write  rst=off  init_reg=0  en=off  latency=2  dbl_ovrd=off  optimize=Area  use_rpm=off  block_type=spram
      settings: xl_area=[0, 0, 0, 0, 0, 0, 0]  block_version=8.2
  dout : Outport  OutDataType=sfix(16)  OutScaling=2^0
  wires:
  din/1 -> Single Port RAM/2
  addr/1 -> Convert2/1
  AddSub2/1 -> Delay5/1
  Constant3/1 -> AddSub2/2
  Single Port RAM/1 -> dout/1
  Delay5/1 -> AddSub2/1, AddSub1/2
  AddSub1/1 -> Single Port RAM/1
  Convert2/1 -> Shift/1
  Shift/1 -> AddSub1/1
  ena/1 -> Delay5/2, Single Port RAM/3

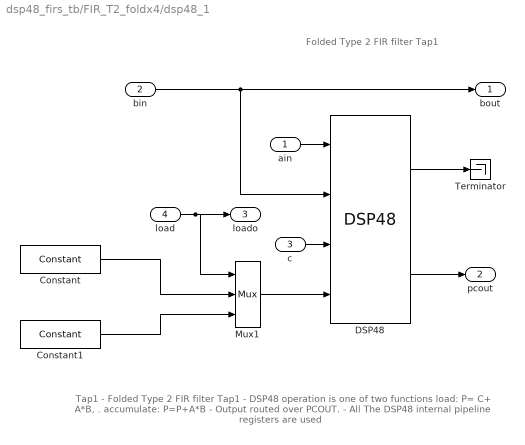
== system dsp48_firs_tb/FIR_T2_foldx4/dsp48_1 ==
  note: Tap1 - Folded Type 2 FIR filter Tap1
      | - DSP48 operation is one of two functions
      |   load:  P= C+ A*B, .
      |   accumulate: P=P+A*B
      | - Output routed over PCOUT.
      | - All The DSP48 internal pipeline registers are used
  note: Folded Type 2 FIR filter Tap1
  ain : Inport  OutDataType=sfix(16)  OutScaling=2^0
  bin : Inport  Port=2  OutDataType=sfix(16)  OutScaling=2^0
  c : Inport  Port=3  OutDataType=sfix(16)  OutScaling=2^0
  load : Inport  Port=4  OutDataType=sfix(16)  OutScaling=2^0
  Constant : xbsIndex_r4/Constant  arith_type=DSP48 Instruction  const=1  n_bits=1  bin_pt=0  explicit_period=off  period=1  equ=P=P+(A*B)  opselect=P + A*B  inp2=PCIN>>17  opr=+  inp1=P  carry=CIN  dbl_ovrd=off  block_type=constant
      settings: block_version=VER_STRING_GOES_HERE
  Constant1 : xbsIndex_r4/Constant  arith_type=DSP48 Instruction  const=1  n_bits=1  bin_pt=0  explicit_period=off  period=1  equ=P=C+(A*B)  opselect=C + A*B  inp2=PCIN>>17  opr=+  inp1=P  carry=CIN  dbl_ovrd=off  block_type=constant
      settings: block_version=VER_STRING_GOES_HERE
  DSP48 : xbsIndex_r4/DSP48  use_b=Direct from B Port  use_op=on  use_creg=on  use_pcin=off  use_pcout=on  use_bcout=off  rst_all=off  en_all=off  pipeline_a=1  pipeline_b=1  pipeline_c=on  pipeline_p=on  pipeline_mult=on  pipeline_opmode=on  pipeline_sub=on  pipeline_carryin=on  pipeline_carryinsel=on  rst_a=off  rst_b=off  rst_c=off  rst_mult=off  rst_p=off  rst_carry_in=off  rst_ctrl=off  en_a=off  en_b=off  en_c=off  en_mult=off  en_p=off  en_carry_in=off  en_ctrl=off  dbl_ovrd=off  use_synth_model=off  xl_useadderonly=off  block_type=dsp48
      settings: xl_use_area=on  xl_area=[0, 0, 0, 0, 0, 0, 0]  block_version=VER_STRING_GOES_HERE
  Mux1 : xbsIndex_r4/Mux  inputs=2  en=off  latency=0  precision=Full  arith_type=Unsigned  n_bits=48  bin_pt=0  quantization=Truncate  overflow=Wrap  dbl_ovrd=off  block_type=mux
      settings: xl_area=[0, 0, 0, 0, 0, 0, 0]  block_version=VER_STRING_GOES_HERE
  Terminator : Terminator
  bout : Outport  OutDataType=sfix(16)  OutScaling=2^0
  pcout : Outport  Port=2  OutDataType=sfix(16)  OutScaling=2^0
  loado : Outport  Port=3  OutDataType=sfix(16)  OutScaling=2^0
  wires:
  load/1 -> Mux1/1, loado/1
  Constant/1 -> Mux1/2
  Constant1/1 -> Mux1/3
  Mux1/1 -> DSP48/4
  ain/1 -> DSP48/1
  bin/1 -> DSP48/2, bout/1
  c/1 -> DSP48/3
  DSP48/2 -> pcout/1
  DSP48/1 -> Terminator/1

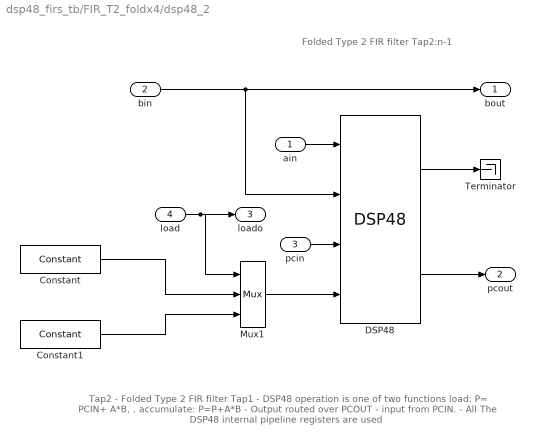
== system dsp48_firs_tb/FIR_T2_foldx4/dsp48_2 ==
  note: Folded Type 2 FIR filter Tap2:n-1
  note: Tap2 - Folded Type 2 FIR filter Tap1
      | - DSP48 operation is one of two functions
      |   load:  P= PCIN+ A*B, .
      |   accumulate: P=P+A*B
      | - Output routed over PCOUT
      | - input from PCIN.
      | - All The DSP48 internal pipeline registers are used
  ain : Inport  OutDataType=sfix(16)  OutScaling=2^0
  bin : Inport  Port=2  OutDataType=sfix(16)  OutScaling=2^0
  pcin : Inport  Port=3  OutDataType=sfix(16)  OutScaling=2^0
  load : Inport  Port=4  OutDataType=sfix(16)  OutScaling=2^0
  Constant : xbsIndex_r4/Constant  arith_type=DSP48 Instruction  const=1  n_bits=1  bin_pt=0  explicit_period=off  period=1  equ=P=P+(A*B)  opselect=P + A*B  inp2=PCIN>>17  opr=+  inp1=P  carry=CIN  dbl_ovrd=off  block_type=constant
      settings: block_version=VER_STRING_GOES_HERE
  Constant1 : xbsIndex_r4/Constant  arith_type=DSP48 Instruction  const=1  n_bits=1  bin_pt=0  explicit_period=off  period=1  equ=P=PCIN+(A*B)  opselect=PCIN + A*B  inp2=PCIN>>17  opr=+  inp1=P  carry=CIN  dbl_ovrd=off  block_type=constant
      settings: block_version=VER_STRING_GOES_HERE
  DSP48 : xbsIndex_r4/DSP48  use_b=Direct from B Port  use_op=on  use_creg=off  use_pcin=on  use_pcout=on  use_bcout=off  rst_all=off  en_all=off  pipeline_a=1  pipeline_b=1  pipeline_c=on  pipeline_p=on  pipeline_mult=on  pipeline_opmode=on  pipeline_sub=on  pipeline_carryin=on  pipeline_carryinsel=on  rst_a=off  rst_b=off  rst_c=off  rst_mult=off  rst_p=off  rst_carry_in=off  rst_ctrl=off  en_a=off  en_b=off  en_c=off  en_mult=off  en_p=off  en_carry_in=off  en_ctrl=off  dbl_ovrd=off  use_synth_model=off  xl_useadderonly=off  block_type=dsp48
      settings: xl_use_area=on  xl_area=[0, 0, 0, 0, 0, 0, 0]  block_version=VER_STRING_GOES_HERE
  Mux1 : xbsIndex_r4/Mux  inputs=2  en=off  latency=0  precision=Full  arith_type=Unsigned  n_bits=48  bin_pt=0  quantization=Truncate  overflow=Wrap  dbl_ovrd=off  block_type=mux
      settings: xl_area=[0, 0, 0, 0, 0, 0, 0]  block_version=VER_STRING_GOES_HERE
  Terminator : Terminator
  bout : Outport  OutDataType=sfix(16)  OutScaling=2^0
  pcout : Outport  Port=2  OutDataType=sfix(16)  OutScaling=2^0
  loado : Outport  Port=3  OutDataType=sfix(16)  OutScaling=2^0
  wires:
  bin/1 -> bout/1, DSP48/2
  ain/1 -> DSP48/1
  Constant1/1 -> Mux1/3
  Constant/1 -> Mux1/2
  load/1 -> loado/1, Mux1/1
  DSP48/2 -> pcout/1
  DSP48/1 -> Terminator/1
  pcin/1 -> DSP48/3
  Mux1/1 -> DSP48/4

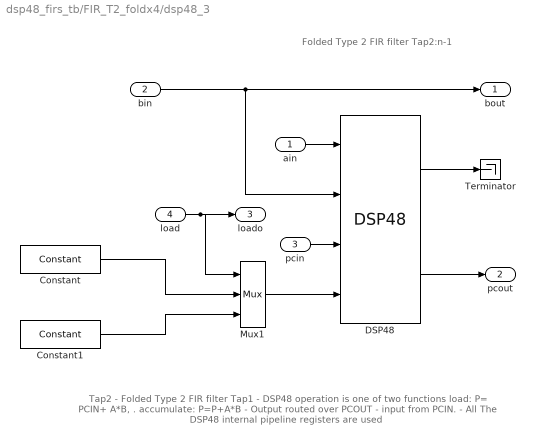
== system dsp48_firs_tb/FIR_T2_foldx4/dsp48_3 ==
  note: Tap2 - Folded Type 2 FIR filter Tap1
      | - DSP48 operation is one of two functions
      |   load:  P= PCIN+ A*B, .
      |   accumulate: P=P+A*B
      | - Output routed over PCOUT
      | - input from PCIN.
      | - All The DSP48 internal pipeline registers are used
  note: Folded Type 2 FIR filter Tap2:n-1
  ain : Inport  OutDataType=sfix(16)  OutScaling=2^0
  bin : Inport  Port=2  OutDataType=sfix(16)  OutScaling=2^0
  pcin : Inport  Port=3  OutDataType=sfix(16)  OutScaling=2^0
  load : Inport  Port=4  OutDataType=sfix(16)  OutScaling=2^0
  Constant : xbsIndex_r4/Constant  arith_type=DSP48 Instruction  const=1  n_bits=1  bin_pt=0  explicit_period=off  period=1  equ=P=P+(A*B)  opselect=P + A*B  inp2=PCIN>>17  opr=+  inp1=P  carry=CIN  dbl_ovrd=off  block_type=constant
      settings: block_version=VER_STRING_GOES_HERE
  Constant1 : xbsIndex_r4/Constant  arith_type=DSP48 Instruction  const=1  n_bits=1  bin_pt=0  explicit_period=off  period=1  equ=P=PCIN+(A*B)  opselect=PCIN + A*B  inp2=PCIN>>17  opr=+  inp1=P  carry=CIN  dbl_ovrd=off  block_type=constant
      settings: block_version=VER_STRING_GOES_HERE
  DSP48 : xbsIndex_r4/DSP48  use_b=Direct from B Port  use_op=on  use_creg=off  use_pcin=on  use_pcout=on  use_bcout=off  rst_all=off  en_all=off  pipeline_a=1  pipeline_b=1  pipeline_c=on  pipeline_p=on  pipeline_mult=on  pipeline_opmode=on  pipeline_sub=on  pipeline_carryin=on  pipeline_carryinsel=on  rst_a=off  rst_b=off  rst_c=off  rst_mult=off  rst_p=off  rst_carry_in=off  rst_ctrl=off  en_a=off  en_b=off  en_c=off  en_mult=off  en_p=off  en_carry_in=off  en_ctrl=off  dbl_ovrd=off  use_synth_model=off  xl_useadderonly=off  block_type=dsp48
      settings: xl_use_area=on  xl_area=[0, 0, 0, 0, 0, 0, 0]  block_version=VER_STRING_GOES_HERE
  Mux1 : xbsIndex_r4/Mux  inputs=2  en=off  latency=0  precision=Full  arith_type=Unsigned  n_bits=48  bin_pt=0  quantization=Truncate  overflow=Wrap  dbl_ovrd=off  block_type=mux
      settings: xl_area=[0, 0, 0, 0, 0, 0, 0]  block_version=VER_STRING_GOES_HERE
  Terminator : Terminator
  bout : Outport  OutDataType=sfix(16)  OutScaling=2^0
  pcout : Outport  Port=2  OutDataType=sfix(16)  OutScaling=2^0
  loado : Outport  Port=3  OutDataType=sfix(16)  OutScaling=2^0
  wires:
  Mux1/1 -> DSP48/4
  pcin/1 -> DSP48/3
  DSP48/1 -> Terminator/1
  DSP48/2 -> pcout/1
  load/1 -> Mux1/1, loado/1
  Constant/1 -> Mux1/2
  Constant1/1 -> Mux1/3
  ain/1 -> DSP48/1
  bin/1 -> DSP48/2, bout/1
